simulink library "csu_tbg_table_based_guidance_lib"  (R2015b)
settings: Solver=ode45  StartTime=0.0  StopTime=10.0  RelTol=1e-3
undefined symbols (not defined in the file or in its folder): DiscIntNeverNeededParam
undefined symbols (not defined in the file): csc_gdn_pwpf_takeoff_hover_translate_table, csc_gdn_pwpf_takeoff_hover_translate_table_length, tlt_terminal_vertical_vel_zero_mean_bias
libraries: simulink x2, util_info_lib x1
settings Model: Creator=mstewart  LastModifiedBy=jimkaidy
settings DataIOCC: SaveFormat=Array
settings DebuggingCC: UnderspecifiedInitializationDetection=Classic  MergeDetectMultiDrivingBlocksExec=none  SolverPrmCheckMsg=warning
settings HardwareCC: ProdBitPerPointer=32  ProdLargestAtomicFloat=None  ProdIntDivRoundTo=Undefined  ProdEndianess=Unspecified  ProdWordSize=32  ProdHWDeviceType=32-bit Generic
settings GRTTargetCC: GeneratePreprocessorConditionals=Disable all
settings ConfigComp: CovModelRefEnable=Off  CovSFcnEnable=off

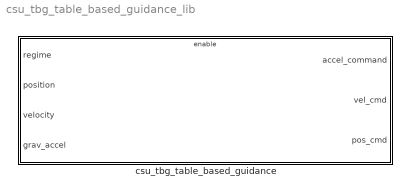
== system csu_tbg_table_based_guidance_lib ==
  csu_tbg_table_based_guidance : Subsystem  mask{guidance_table=csc_gdn_pwpf_takeoff_hover_translate_table, guidance_table_num_entries=csc_gdn_pwpf_takeoff_hover_translate_table_length, entry_comparison=>=, velocity_bias=[0 0 tlt_terminal_vertical_vel_zero_mean_bias]}
      mask prompts: guidance_table "Guidance Table"; guidance_table_num_entries "Number of Entries in Table"; entry_comparison "Entry Comparison"; velocity_bias "Commanded Velocity Bias"
      mask init:
      | csu_tbg_table_based_guidance_callback(gcb, entry_comparison);
      mask TypeOptions entry_comparison: >= | <
      mask Display:
      | mask_values = get_param(gcb,'MaskValues');
      | disp(['Table Guidance:\n' mask_values{1}]);

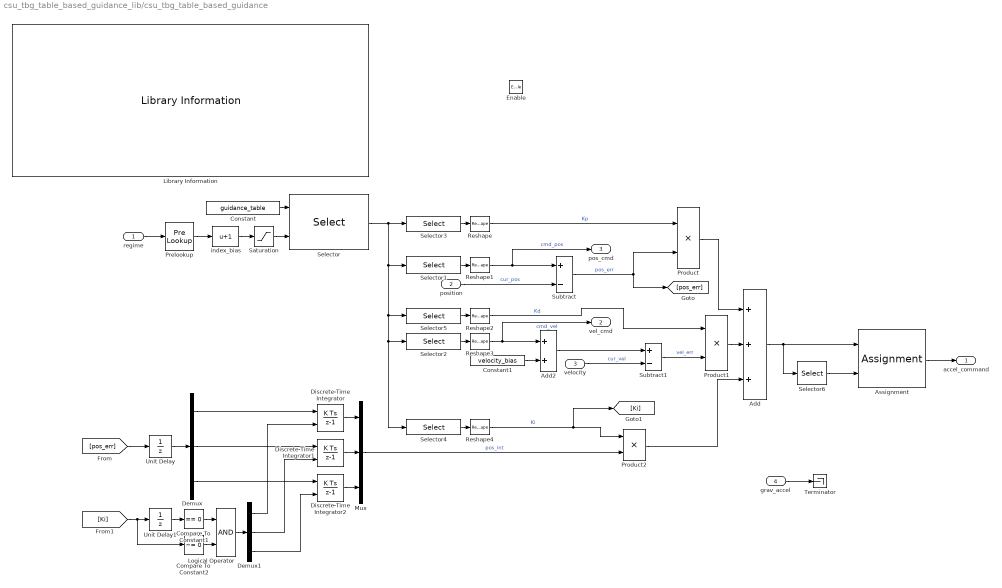
== system csu_tbg_table_based_guidance_lib/csu_tbg_table_based_guidance ==
  regime : Inport
  position : Inport  Port=2
  velocity : Inport  Port=3
  grav_accel : Inport  Port=4
  Enable : EnablePort
  Add : Sum  Inputs=+++  InputSameDT=on
  Add2 : Sum
  Assignment : Assignment  IndexOptions=Index vector (dialog)  Indices=3  OutputSizes=1
  Compare To Constant1 : simulink/Logic and Bit Operations/Compare To Constant  relop===  const=0  OutDataTypeStr=boolean
  Compare To Constant2 : simulink/Logic and Bit Operations/Compare To Constant  relop=~=  const=0  OutDataTypeStr=boolean
  Constant : Constant  Value=guidance_table
  Constant1 : Constant  Value=velocity_bias
  Demux : Demux  Outputs=3
  Demux1 : Demux  Outputs=3
  Discrete-Time Integrator : DiscreteIntegrator  ExternalReset=rising  SampleTime=-1  ICPrevOutput=DiscIntNeverNeededParam  ICPrevScaledInput=DiscIntNeverNeededParam
  Discrete-Time Integrator1 : DiscreteIntegrator  ExternalReset=rising  SampleTime=-1  ICPrevOutput=DiscIntNeverNeededParam  ICPrevScaledInput=DiscIntNeverNeededParam
  Discrete-Time Integrator2 : DiscreteIntegrator  ExternalReset=rising  SampleTime=-1  ICPrevOutput=DiscIntNeverNeededParam  ICPrevScaledInput=DiscIntNeverNeededParam
  Library Information : util_info_lib/Library Information  owner='NONE'
  Logical Operator : Logic  AllPortsSameDT=off  OutDataTypeStr=boolean
  Mux : Mux  Inputs=3
  Prelookup : PreLookup  BreakpointsData=guidance_table(:,1)  BeginIndexSearchUsingPreviousIndexResult=on  OutputOnlyTheIndex=on
  Product : Product  InputSameDT=on
  Product1 : Product  InputSameDT=on
  Product2 : Product  InputSameDT=on
  Reshape{,1..4} (5 alike) : Reshape
  Saturation : Saturate  UpperLimit=guidance_table_num_entries  LowerLimit=1
  Selector : Selector  NumberOfDimensions=2  InputPortWidth=3  IndexOptions=Index vector (port),Select all  Indices=[1 3],1  OutputSizes=1,1
  Selector1 : Selector  InputPortWidth=16  IndexOptions=Index vector (dialog)  Indices=tbg_cmd_pos_indices  OutputSizes=1
  Selector2 : Selector  InputPortWidth=16  IndexOptions=Index vector (dialog)  Indices=tbg_cmd_vel_indices  OutputSizes=1
  Selector3 : Selector  InputPortWidth=16  IndexOptions=Index vector (dialog)  Indices=tbg_kp_indices  OutputSizes=1
  Selector4 : Selector  InputPortWidth=16  IndexOptions=Index vector (dialog)  Indices=tbg_ki_indices  OutputSizes=1
  Selector5 : Selector  InputPortWidth=16  IndexOptions=Index vector (dialog)  Indices=tbg_kd_indices  OutputSizes=1
  Selector6 : Selector  InputPortWidth=3  IndexOptions=Index vector (dialog)  Indices=3  OutputSizes=1
  Subtract : Sum  Inputs=+-
  Subtract1 : Sum  Inputs=+-
  Terminator : Terminator
  Unit Delay : UnitDelay  SampleTime=-1
  Unit Delay1 : UnitDelay  SampleTime=-1
  index_bias : Bias  Bias=1
  accel_command : Outport
  vel_cmd : Outport  Port=2
  pos_cmd : Outport  Port=3
  wires:
  Add2/1 -> Subtract1/1
  Logical Operator/1 -> Demux1/1
  Compare To Constant2/1 -> Logical Operator/2
  Demux1/1 -> Discrete-Time Integrator/2
  Demux1/3 -> Discrete-Time Integrator2/2
  Demux1/2 -> Discrete-Time Integrator1/2
  Compare To Constant1/1 -> Logical Operator/1
  Unit Delay1/1 -> Compare To Constant1/1
  [Ki] -> Unit Delay1/1, Compare To Constant2/1
  Discrete-Time Integrator2/1 -> Mux/3
  Discrete-Time Integrator1/1 -> Mux/2
  Discrete-Time Integrator/1 -> Mux/1
  Unit Delay/1 -> Demux/1
  Demux/3 -> Discrete-Time Integrator2/1
  Demux/2 -> Discrete-Time Integrator1/1
  Demux/1 -> Discrete-Time Integrator/1
  [pos_err] -> Unit Delay/1
  Assignment/1 -> accel_command/1
  Add/1 -> Selector6/1, Assignment/1
  grav_accel/1 -> Terminator/1
  Product2/1 -> Add/3
  Mux/1 -> Product2/2  "pos_int"
  Product1/1 -> Add/2
  Product/1 -> Add/1
  Subtract1/1 -> Product1/2  "vel_err"
  Subtract/1 -> Product/2, [pos_err]  "pos_err"
  position/1 -> Subtract/2  "cur_pos"
  Selector5/1 -> Reshape2/1
  Selector3/1 -> Reshape/1
  Selector4/1 -> Reshape4/1
  Selector/1 -> Selector3/1, Selector1/1, Selector5/1, Selector2/1, Selector4/1
  Selector2/1 -> Reshape3/1
  Selector1/1 -> Reshape1/1
  index_bias/1 -> Saturation/1
  Constant/1 -> Selector/1
  Prelookup/1 -> index_bias/1
  regime/1 -> Prelookup/1
  Reshape/1 -> Product/1  "Kp"
  Reshape1/1 -> pos_cmd/1, Subtract/1  "cmd_pos"
  Reshape2/1 -> Product1/1  "Kd"
  Reshape3/1 -> vel_cmd/1, Add2/1  "cmd_vel"
  Reshape4/1 -> Product2/1, [Ki]  "Ki"
  velocity/1 -> Subtract1/2  "cur_vel"
  Constant1/1 -> Add2/2
  Saturation/1 -> Selector/2
  Selector6/1 -> Assignment/2
